simulink model "lqg_model"  (R2024a)
settings: Solver=FixedStepAuto  StartTime=0.0  StopTime=5  FixedStep=0.0001  RelTol=1e-3
values from neighbouring files (symbols this model uses):
  A = [20 5 -16 9; 6 1 -4 1; 32 9 -25 14; 8 4 -6 4]    [lqe.m]    (also in lqg.m = [5 -5 -9 3; -5 5 -3 9; -9 -3 5 5; 3 9 5 5]; lqr.m = [11 -2 13; 6 -1 6; -6 -1 -8])
  B = [2 0; 6 0; 6 0; 2 0]    [lqg.m]    (also in lqr.m = [2; 0; 0])
  C = [-1 0 1 -1]    [lqe.m]    (also in lqg.m = [1 -1 1 1; 1 3 -1 3])
  D = [0 2; 0 1]    [lqg.m]
  K = -Rk\B'*Pk    [lqg.m]
  L = L1    [lqe.m]    (also in lqg.m = -Pl*C'/Rl)
  x0 = [1; 1; 1; 1]    [lqe.m]    (also in lqg.m; lqr.m = [1; 1; 1])
  xhat0 = [0; 0; 0; 0]    [lqg.m]
settings Model: Creator=ventus  LastModifiedBy=ventus

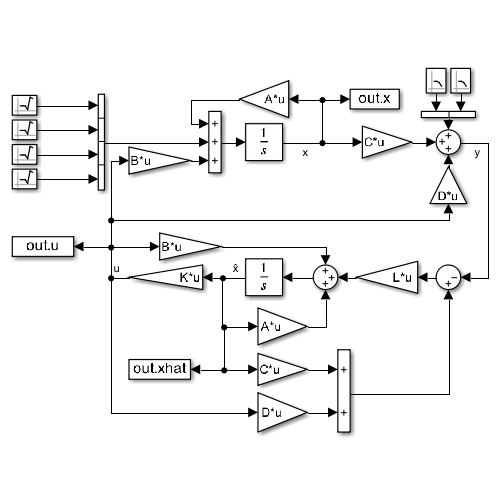
[thumbnail: Simulink's stored preview of the top-level diagram]
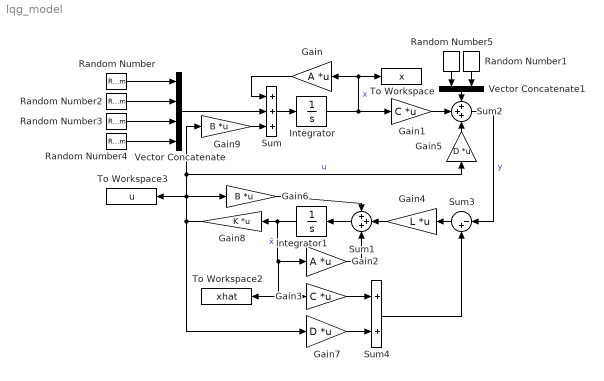
== system lqg_model ==
  Gain : Gain  Gain=A  Multiplication=Matrix(K*u)
  Gain1 : Gain  Gain=C  Multiplication=Matrix(K*u)
  Gain2 : Gain  Gain=A  Multiplication=Matrix(K*u)
  Gain3 : Gain  Gain=C  Multiplication=Matrix(K*u)
  Gain4 : Gain  Gain=L  Multiplication=Matrix(K*u)
  Gain5 : Gain  Gain=D  Multiplication=Matrix(K*u)
  Gain6 : Gain  Gain=B  Multiplication=Matrix(K*u)
  Gain7 : Gain  Gain=D  Multiplication=Matrix(K*u)
  Gain8 : Gain  Gain=K  Multiplication=Matrix(K*u)
  Gain9 : Gain  Gain=B  Multiplication=Matrix(K*u)
  Integrator : Integrator  InitialCondition=x0
  Integrator1 : Integrator  InitialCondition=xhat0
  Random Number : RandomNumber  SampleTime=0  VectorParams1D=off
  Random Number1 : RandomNumber  Variance=5  Seed=5  SampleTime=0  VectorParams1D=off
  Random Number2 : RandomNumber  Variance=2  Seed=1  SampleTime=0  VectorParams1D=off
  Random Number3 : RandomNumber  Variance=4  Seed=2  SampleTime=0  VectorParams1D=off
  Random Number4 : RandomNumber  Variance=3  Seed=3  SampleTime=0  VectorParams1D=off
  Random Number5 : RandomNumber  Variance=2  Seed=4  SampleTime=0  VectorParams1D=off
  Sum : Sum  Inputs=+++
  Sum1 : Sum  Inputs=+++
  Sum2 : Sum  Inputs=+++
  Sum3 : Sum  Inputs=|-+
  Sum4 : Sum
  To Workspace : ToWorkspace  VariableName=x  SaveFormat=Timeseries  SampleTime=-1
  To Workspace2 : ToWorkspace  VariableName=xhat  SaveFormat=Timeseries  SampleTime=-1
  To Workspace3 : ToWorkspace  VariableName=u  SaveFormat=Timeseries  SampleTime=-1
  Vector Concatenate : Concatenate  NumInputs=4
  Vector Concatenate1 : Concatenate
  wires:
  Gain4/1 -> Sum1/2
  Sum3/1 -> Gain4/1
  Gain/1 -> Sum/1
  Integrator1/1 -> Gain3/1, To Workspace2/1, Gain2/1, Gain8/1  "x̂"
  Sum2/1 -> Sum3/1  "y"
  Sum1/1 -> Integrator1/1
  Gain2/1 -> Sum1/3
  Sum/1 -> Integrator/1
  Integrator/1 -> Gain1/1, Gain/1, To Workspace/1  "x"
  Gain1/1 -> Sum2/2
  Gain8/1 -> Gain7/1, Gain6/1, Gain5/1, Gain9/1, To Workspace3/1  "u"
  Gain9/1 -> Sum/3
  Gain5/1 -> Sum2/3
  Random Number/1 -> Vector Concatenate/1
  Random Number3/1 -> Vector Concatenate/3
  Random Number4/1 -> Vector Concatenate/4
  Random Number2/1 -> Vector Concatenate/2
  Vector Concatenate/1 -> Sum/2
  Random Number5/1 -> Vector Concatenate1/1
  Random Number1/1 -> Vector Concatenate1/2
  Vector Concatenate1/1 -> Sum2/1
  Gain6/1 -> Sum1/1
  Gain3/1 -> Sum4/1
  Gain7/1 -> Sum4/2
  Sum4/1 -> Sum3/2
